simulink model "Modelo_inicial"  (R2021b)
settings: Solver=ode23tb  StartTime=0.0  StopTime=10  RelTol=1e-3
values from neighbouring files (symbols this model uses):
  A1 = 1.2566e-3    (= 0.0012566)    [modelo_inicial.m]
  A2 = 8.765e-4    (= 0.0008765)    [modelo_inicial.m]
  be = 9000e5    (= 900000000)    [modelo_inicial.m]
  f = 1500    [modelo_inicial.m]
  g = 9.8    [modelo_inicial.m]
  kc1 = 3.644e-12    [modelo_inicial.m]
  kc2 = 4.376e-12    [modelo_inicial.m]
  kq1 = 4.76e-4    (= 0.000476)    [modelo_inicial.m]
  kq2 = 4.76e-4    (= 0.000476)    [modelo_inicial.m]
  M = 84    [modelo_inicial.m]
  V1 = VL1+(A1*xe0)    (= 0.0001330412)    [modelo_inicial.m]
  V2 = VL2+A2*(L-xe0)    (= 0.000153427)    [modelo_inicial.m]
libraries: simulink x1
settings Model: Creator=cof_2  LastModifiedBy=cof_2

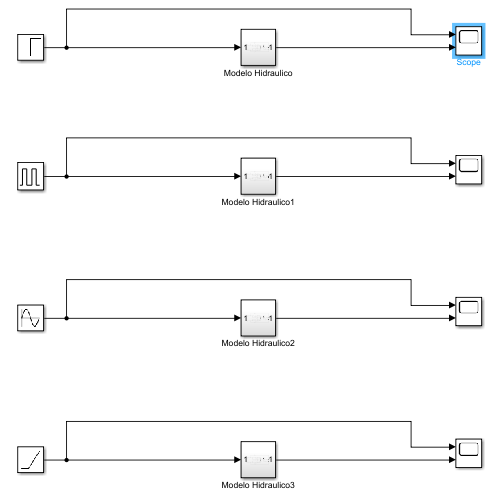
[thumbnail: Simulink's stored preview of the top-level diagram]
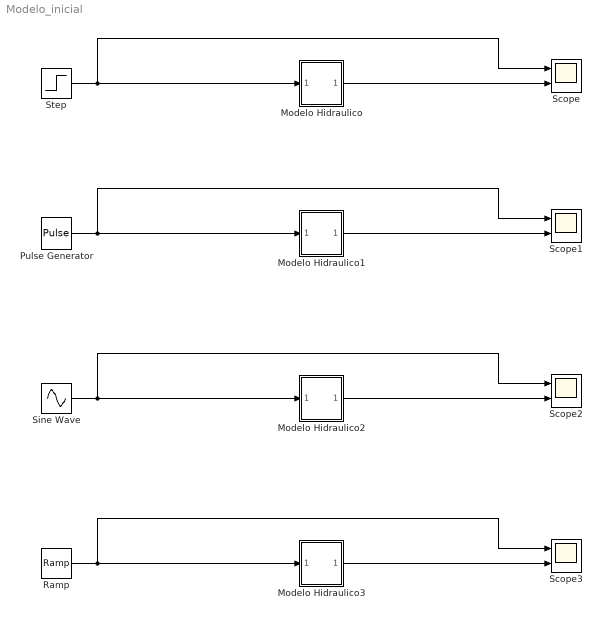
== system Modelo_inicial ==
  Modelo Hidraulico : Subsystem
  Modelo Hidraulico1 : Subsystem
  Modelo Hidraulico2 : Subsystem
  Modelo Hidraulico3 : Subsystem
  Pulse Generator : DiscretePulseGenerator  PulseType=Time based  Period=2.5  PulseWidth=5
  Ramp : simulink/Sources/Ramp  slope=1  start=0  InitialOutput=0
  Scope{,1..3} (4 alike) : Scope  NumInputPorts=2
  Sine Wave : Sin  SampleTime=0
  Step : Step  SampleTime=0
  wires:
  Modelo Hidraulico/1(Out1) -> Scope/2
  Step/1 -> Modelo Hidraulico/1(In1), Scope/1
  Pulse Generator/1 -> Scope1/1, Modelo Hidraulico1/1(In1)
  Modelo Hidraulico1/1(Out1) -> Scope1/2
  Sine Wave/1 -> Modelo Hidraulico2/1(In1), Scope2/1
  Modelo Hidraulico2/1(Out1) -> Scope2/2
  Ramp/1 -> Modelo Hidraulico3/1(In1), Scope3/1
  Modelo Hidraulico3/1(Out1) -> Scope3/2

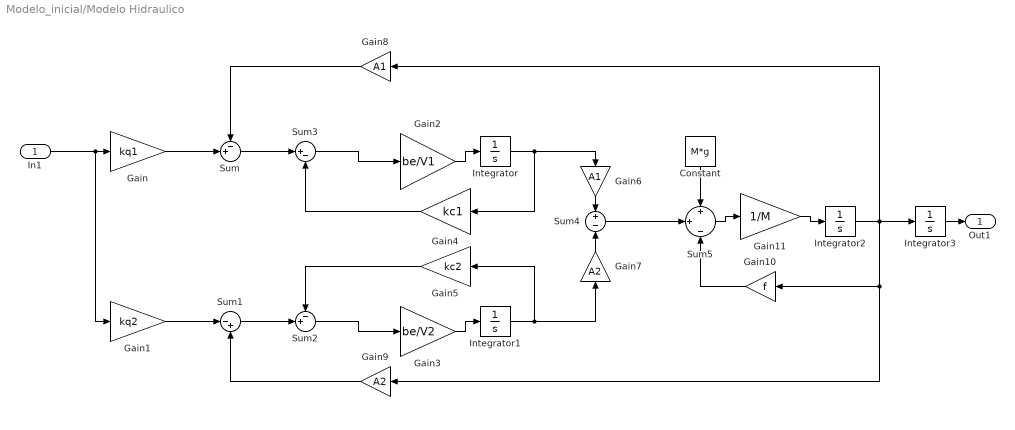
== system Modelo_inicial/Modelo Hidraulico ==
  In1 : Inport
  Constant : Constant  Value=M*g
  Gain : Gain  Gain=kq1
  Gain1 : Gain  Gain=kq2
  Gain10 : Gain  Gain=f
  Gain11 : Gain  Gain=1/M
  Gain2 : Gain  Gain=be/V1
  Gain3 : Gain  Gain=be/V2
  Gain4 : Gain  Gain=kc1
  Gain5 : Gain  Gain=kc2
  Gain6 : Gain  Gain=A1
  Gain7 : Gain  Gain=A2
  Gain8 : Gain  Gain=A1
  Gain9 : Gain  Gain=A2
  Integrator{,1..3} (4 alike) : Integrator
  Sum : Sum  Inputs=-+|
  Sum1 : Sum  Inputs=|-+
  Sum2 : Sum  Inputs=-+|
  Sum3 : Sum  Inputs=|+-
  Sum4 : Sum  Inputs=+|-
  Sum5 : Sum  Inputs=+|+|-
  Out1 : Outport
  wires:
  Sum/1 -> Sum3/1
  Constant/1 -> Sum5/1
  Sum4/1 -> Sum5/2
  Gain6/1 -> Sum4/1
  Integrator1/1 -> Gain7/1, Gain5/1
  Gain1/1 -> Sum1/1
  Integrator/1 -> Gain6/1, Gain4/1
  Sum1/1 -> Sum2/2
  Gain2/1 -> Integrator/1
  Sum5/1 -> Gain11/1
  Gain7/1 -> Sum4/2
  Gain/1 -> Sum/2
  Gain8/1 -> Sum/1
  Sum3/1 -> Gain2/1
  Integrator2/1 -> Gain8/1, Integrator3/1, Gain9/1, Gain10/1
  Gain10/1 -> Sum5/3
  Sum2/1 -> Gain3/1
  Gain5/1 -> Sum2/1
  Gain4/1 -> Sum3/2
  Gain3/1 -> Integrator1/1
  Gain9/1 -> Sum1/2
  Gain11/1 -> Integrator2/1
  In1/1 -> Gain1/1, Gain/1
  Integrator3/1 -> Out1/1

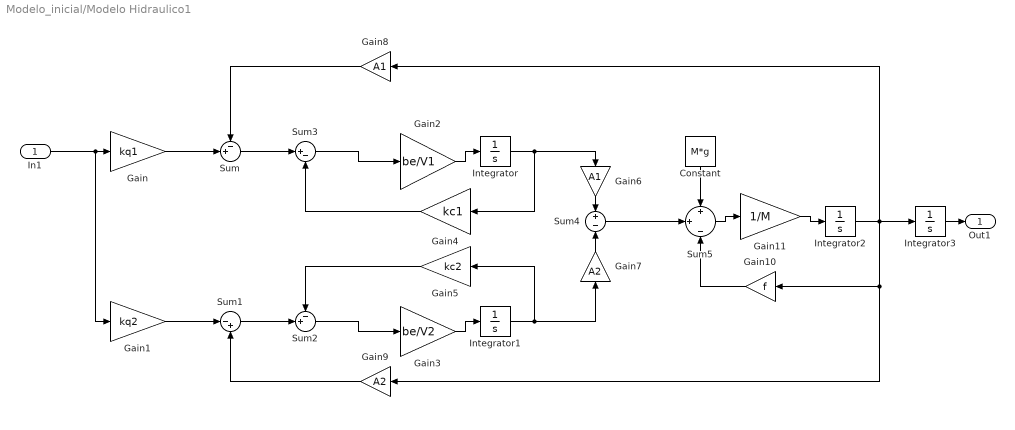
== system Modelo_inicial/Modelo Hidraulico1 ==
  In1 : Inport
  Constant : Constant  Value=M*g
  Gain : Gain  Gain=kq1
  Gain1 : Gain  Gain=kq2
  Gain10 : Gain  Gain=f
  Gain11 : Gain  Gain=1/M
  Gain2 : Gain  Gain=be/V1
  Gain3 : Gain  Gain=be/V2
  Gain4 : Gain  Gain=kc1
  Gain5 : Gain  Gain=kc2
  Gain6 : Gain  Gain=A1
  Gain7 : Gain  Gain=A2
  Gain8 : Gain  Gain=A1
  Gain9 : Gain  Gain=A2
  Integrator{,1..3} (4 alike) : Integrator
  Sum : Sum  Inputs=-+|
  Sum1 : Sum  Inputs=|-+
  Sum2 : Sum  Inputs=-+|
  Sum3 : Sum  Inputs=|+-
  Sum4 : Sum  Inputs=+|-
  Sum5 : Sum  Inputs=+|+|-
  Out1 : Outport
  wires:
  Sum/1 -> Sum3/1
  Constant/1 -> Sum5/1
  Sum4/1 -> Sum5/2
  Gain6/1 -> Sum4/1
  Integrator1/1 -> Gain7/1, Gain5/1
  Gain1/1 -> Sum1/1
  Integrator/1 -> Gain6/1, Gain4/1
  Sum1/1 -> Sum2/2
  Gain2/1 -> Integrator/1
  Sum5/1 -> Gain11/1
  Gain7/1 -> Sum4/2
  Gain/1 -> Sum/2
  Gain8/1 -> Sum/1
  Sum3/1 -> Gain2/1
  Integrator2/1 -> Gain8/1, Integrator3/1, Gain9/1, Gain10/1
  Gain10/1 -> Sum5/3
  Sum2/1 -> Gain3/1
  Gain5/1 -> Sum2/1
  Gain4/1 -> Sum3/2
  Gain3/1 -> Integrator1/1
  Gain9/1 -> Sum1/2
  Gain11/1 -> Integrator2/1
  In1/1 -> Gain1/1, Gain/1
  Integrator3/1 -> Out1/1

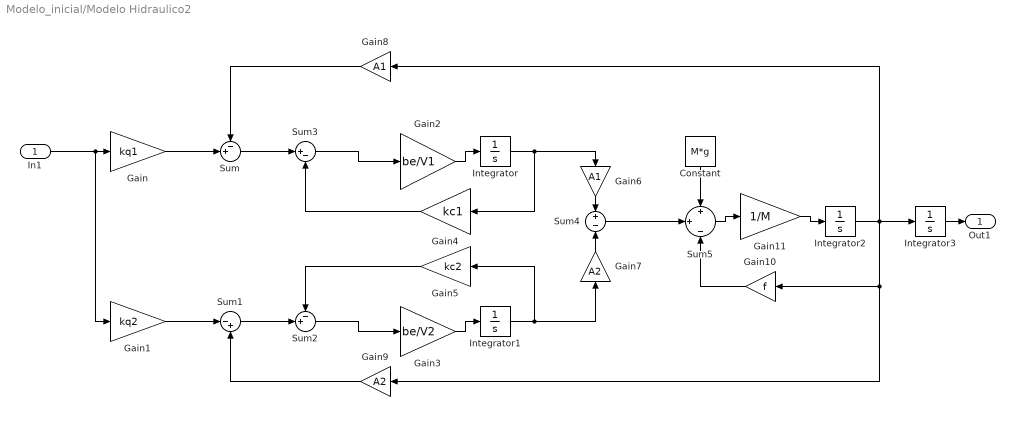
== system Modelo_inicial/Modelo Hidraulico2 ==
  In1 : Inport
  Constant : Constant  Value=M*g
  Gain : Gain  Gain=kq1
  Gain1 : Gain  Gain=kq2
  Gain10 : Gain  Gain=f
  Gain11 : Gain  Gain=1/M
  Gain2 : Gain  Gain=be/V1
  Gain3 : Gain  Gain=be/V2
  Gain4 : Gain  Gain=kc1
  Gain5 : Gain  Gain=kc2
  Gain6 : Gain  Gain=A1
  Gain7 : Gain  Gain=A2
  Gain8 : Gain  Gain=A1
  Gain9 : Gain  Gain=A2
  Integrator{,1..3} (4 alike) : Integrator
  Sum : Sum  Inputs=-+|
  Sum1 : Sum  Inputs=|-+
  Sum2 : Sum  Inputs=-+|
  Sum3 : Sum  Inputs=|+-
  Sum4 : Sum  Inputs=+|-
  Sum5 : Sum  Inputs=+|+|-
  Out1 : Outport
  wires:
  Sum/1 -> Sum3/1
  Constant/1 -> Sum5/1
  Sum4/1 -> Sum5/2
  Gain6/1 -> Sum4/1
  Integrator1/1 -> Gain7/1, Gain5/1
  Gain1/1 -> Sum1/1
  Integrator/1 -> Gain6/1, Gain4/1
  Sum1/1 -> Sum2/2
  Gain2/1 -> Integrator/1
  Sum5/1 -> Gain11/1
  Gain7/1 -> Sum4/2
  Gain/1 -> Sum/2
  Gain8/1 -> Sum/1
  Sum3/1 -> Gain2/1
  Integrator2/1 -> Gain8/1, Integrator3/1, Gain9/1, Gain10/1
  Gain10/1 -> Sum5/3
  Sum2/1 -> Gain3/1
  Gain5/1 -> Sum2/1
  Gain4/1 -> Sum3/2
  Gain3/1 -> Integrator1/1
  Gain9/1 -> Sum1/2
  Gain11/1 -> Integrator2/1
  In1/1 -> Gain1/1, Gain/1
  Integrator3/1 -> Out1/1

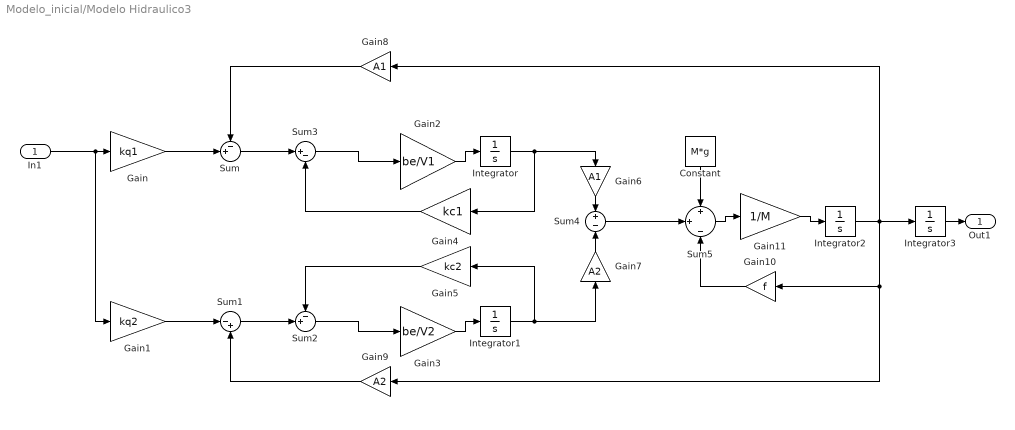
== system Modelo_inicial/Modelo Hidraulico3 ==
  In1 : Inport
  Constant : Constant  Value=M*g
  Gain : Gain  Gain=kq1
  Gain1 : Gain  Gain=kq2
  Gain10 : Gain  Gain=f
  Gain11 : Gain  Gain=1/M
  Gain2 : Gain  Gain=be/V1
  Gain3 : Gain  Gain=be/V2
  Gain4 : Gain  Gain=kc1
  Gain5 : Gain  Gain=kc2
  Gain6 : Gain  Gain=A1
  Gain7 : Gain  Gain=A2
  Gain8 : Gain  Gain=A1
  Gain9 : Gain  Gain=A2
  Integrator{,1..3} (4 alike) : Integrator
  Sum : Sum  Inputs=-+|
  Sum1 : Sum  Inputs=|-+
  Sum2 : Sum  Inputs=-+|
  Sum3 : Sum  Inputs=|+-
  Sum4 : Sum  Inputs=+|-
  Sum5 : Sum  Inputs=+|+|-
  Out1 : Outport
  wires:
  Sum/1 -> Sum3/1
  Constant/1 -> Sum5/1
  Sum4/1 -> Sum5/2
  Gain6/1 -> Sum4/1
  Integrator1/1 -> Gain7/1, Gain5/1
  Gain1/1 -> Sum1/1
  Integrator/1 -> Gain6/1, Gain4/1
  Sum1/1 -> Sum2/2
  Gain2/1 -> Integrator/1
  Sum5/1 -> Gain11/1
  Gain7/1 -> Sum4/2
  Gain/1 -> Sum/2
  Gain8/1 -> Sum/1
  Sum3/1 -> Gain2/1
  Integrator2/1 -> Gain8/1, Integrator3/1, Gain9/1, Gain10/1
  Gain10/1 -> Sum5/3
  Sum2/1 -> Gain3/1
  Gain5/1 -> Sum2/1
  Gain4/1 -> Sum3/2
  Gain3/1 -> Integrator1/1
  Gain9/1 -> Sum1/2
  Gain11/1 -> Integrator2/1
  In1/1 -> Gain1/1, Gain/1
  Integrator3/1 -> Out1/1
